simulink model "FirstOrderModelComposite"  (R2021b)
settings: Solver=VariableStepAuto  StartTime=0.0  StopTime=50  RelTol=1e-3
undefined symbols (not defined in the file): delay1, delay2, k, tau
settings Model: Creator=Jonah  LastModifiedBy=Jonah

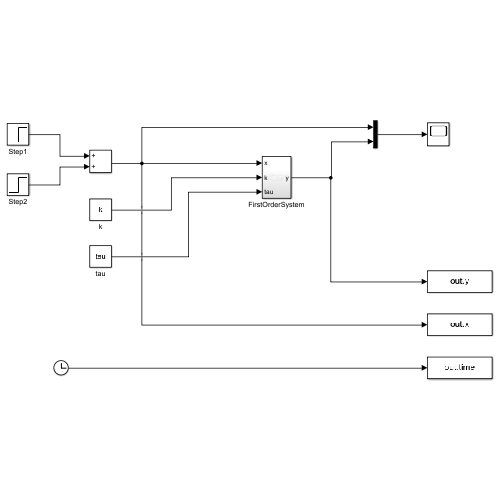
[thumbnail: Simulink's stored preview of the top-level diagram]
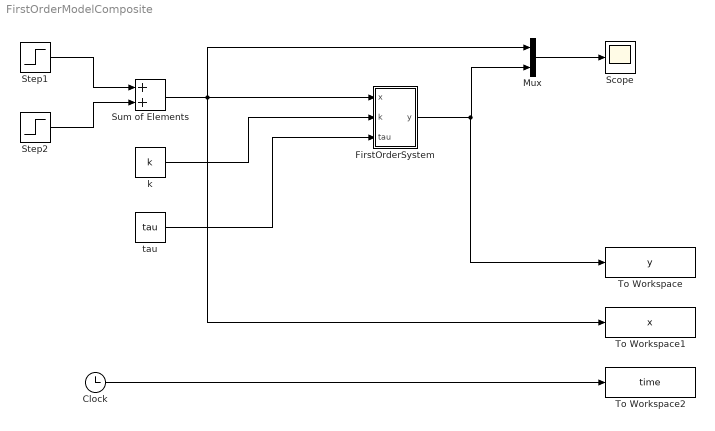
== system FirstOrderModelComposite ==
  Clock : Clock
  FirstOrderSystem : Subsystem
  Mux : Mux  Inputs=2
  Scope : Scope
  Step1 : Step  Time=delay1  SampleTime=0
  Step2 : Step  Time=delay2  SampleTime=0
  Sum of Elements : Sum
  To Workspace : ToWorkspace  VariableName=y  SampleTime=-1
  To Workspace1 : ToWorkspace  VariableName=x  SampleTime=-1
  To Workspace2 : ToWorkspace  VariableName=time  SampleTime=-1
  k : Constant  Value=k
  tau : Constant  Value=tau
  wires:
  Clock/1 -> To Workspace2/1
  FirstOrderSystem/1(y) -> To Workspace/1, Mux/2
  Mux/1 -> Scope/1
  k/1 -> FirstOrderSystem/2(k)
  Sum of Elements/1 -> To Workspace1/1, Mux/1, FirstOrderSystem/1(x)
  tau/1 -> FirstOrderSystem/3(tau)
  Step2/1 -> Sum of Elements/2
  Step1/1 -> Sum of Elements/1

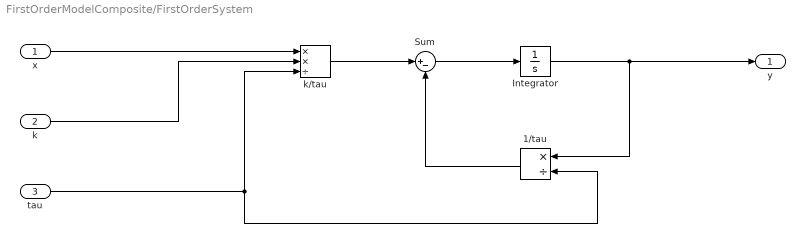
== system FirstOrderModelComposite/FirstOrderSystem ==
  x : Inport
  k : Inport  Port=2
  tau : Inport  Port=3
  1/tau : Product  Inputs=*/
  Integrator : Integrator
  Sum : Sum  Inputs=|+-
  k/tau : Product  Inputs=**/
  y : Outport
  wires:
  Integrator/1 -> y/1, 1/tau/1
  tau/1 -> k/tau/3, 1/tau/2
  Sum/1 -> Integrator/1
  1/tau/1 -> Sum/2
  k/1 -> k/tau/2
  k/tau/1 -> Sum/1
  x/1 -> k/tau/1
